simulink model "Inverter_Three_Phase_Pulses"  (R2021a)
settings: Solver=VariableStepAuto  StartTime=0.0  StopTime=1/60  RelTol=1e-3
libraries: spspowerguiLib x1
settings Model: Creator=Pichau  LastModifiedBy=Pichau

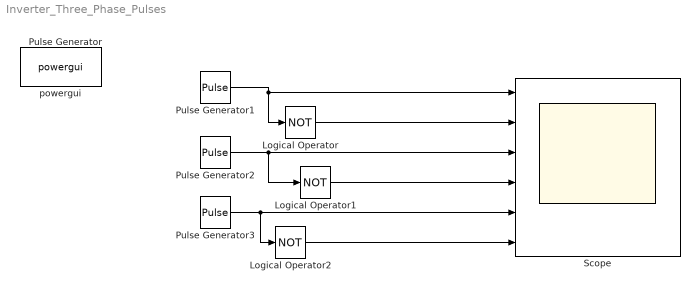
== system Inverter_Three_Phase_Pulses ==
  Logical Operator : Logic  Operator=NOT  AllPortsSameDT=off  OutDataTypeStr=boolean
  Logical Operator1 : Logic  Operator=NOT  AllPortsSameDT=off  OutDataTypeStr=boolean
  Logical Operator2 : Logic  Operator=NOT  AllPortsSameDT=off  OutDataTypeStr=boolean
  Pulse Generator : DiscretePulseGenerator  PulseType=Time based  Period=10  PulseWidth=5
  Pulse Generator1 : DiscretePulseGenerator  PulseType=Time based  Period=1/60  PulseWidth=50
  Pulse Generator2 : DiscretePulseGenerator  PulseType=Time based  Period=1/60  PulseWidth=50  PhaseDelay=-240/360*(1/60)
  Pulse Generator3 : DiscretePulseGenerator  PulseType=Time based  Period=1/60  PulseWidth=50  PhaseDelay=-120/360*(1/60)
  Scope : Scope  NumInputPorts=6
  powergui : spspowerguiLib/powergui  Priority=1  SimulationMode=Continuous  SampleTime=50e-6  frequency=60  Iterations=50  frequencyindice=60  Pbase=100e6  ErrMax=1e-4  UnitsV=kV  UnitsW=MW  buscounter=0  FunctionMessages=off  echomessages=off  EnableUseOfTLC=off  CurrentSourceSwitches=off  DisableSnubberDevices=off  DisableRonSwitches=off  DisableVfSwitches=off  DisplayEquations=off  AutomaticDiscreteSolvers=off  SolverType=Tustin/Backward Euler (TBE)  Interpol=off  ExternalGateDelay=off  methode=off  Ts=100  x0status=blocks  SPID=on  SwTol=0  HookPort=off  NonlinearTolerance=1e-4  nMaxIteration=100  ContinueOnMaxIteration=off  RestoreLinks=warning  ResistiveCurrentMeasurement=off  Frange=[0:2:500]  Ylog=off  Xlog=on  ShowGrid=off  save=off  variable=ZData  structure=0  ZoomFFT=off  StartTime=0.0  cycles=1  DisplayStyle=1  fundamental=60  FreqAxis=off  MaxFrequency=1000  frequencyindicesteady=1  RmsSteady=1  display=off
  wires:
  Pulse Generator1/1 -> Logical Operator/1, Scope/1
  Logical Operator/1 -> Scope/2
  Logical Operator1/1 -> Scope/4
  Pulse Generator2/1 -> Logical Operator1/1, Scope/3
  Pulse Generator3/1 -> Logical Operator2/1, Scope/5
  Logical Operator2/1 -> Scope/6
